simulink model "combined_uc_battery_model"  (R2020a)
settings: Solver=VariableStepAuto  StartTime=0.0  StopTime=3600  RelTol=1e-3
values from neighbouring files (symbols this model uses):
  AH = Q/Vnom    (= 100)    [combined_uc_lion.m]
  Ri = 0.001    [combined_uc_lion.m]
  SOC0 = 0.5    [combined_uc_lion.m]
undefined symbols (not defined in the file or in its folder): DiscIntNeverNeededParam
libraries: fl_lib x5, nesl_utility x4, ee_lib x3
settings Model: Creator=sateeshk  LastModifiedBy=sateeshk

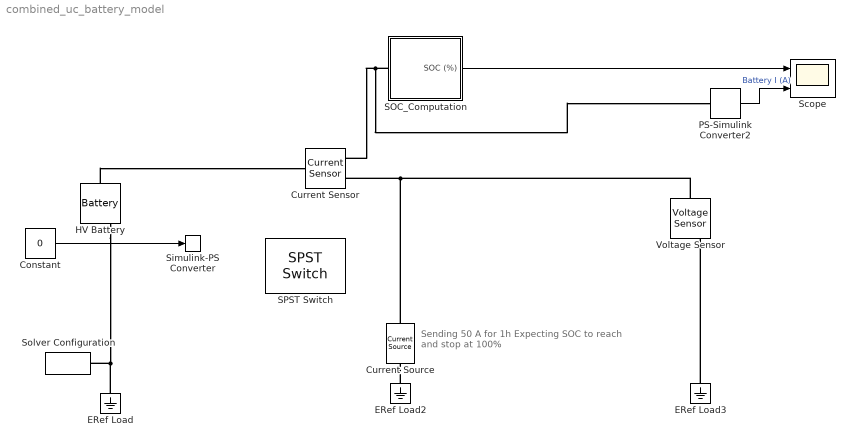
== system combined_uc_battery_model ==
  note: Sending 50 A for 1h
      | Expecting SOC to reach and stop at 100%
  Constant : Constant  Value=0
  Current Sensor : fl_lib/Electrical/Electrical Sensors/Current Sensor
  Current Source : ee_lib/Sources/Current Source  dc_current=50 A  ac_current=0 A  ac_shift=0 rad  ac_frequency=0 Hz  noise_mode=0  PSD=0 A^2/Hz  repeatability=1  auto_seed=4251803758  user_seed=0  sample_time=1e-3 s  i_specify=off  i_priority=None  i=0 A  i_nominal_specify=off  i_nominal_unit=A  i_nominal_value=1  v_specify=off  v_priority=None  v=0 V  v_nominal_specify=off  v_nominal_unit=V  v_nominal_value=1
      settings: SourceProductBaseCode=PS
  ERef Load : fl_lib/Electrical/Electrical Elements/Electrical Reference
      settings: SourceProductBaseCode=MT,SS
  ERef Load2 : fl_lib/Electrical/Electrical Elements/Electrical Reference
      settings: SourceProductBaseCode=MT,SS
  ERef Load3 : fl_lib/Electrical/Electrical Elements/Electrical Reference
      settings: SourceProductBaseCode=MT,SS
  HV Battery : ee_lib/Sources/Battery  Vnom=Vnom V  R1=Ri Ohm  prm_AH=2  AH=AH hr*A  V1=V1 V  AH1=AH1 hr*A  prm_R2=1  R2=2000 Ohm  prm_dyn=1  Rp1=0.005 Ohm  tau1=30 s  Rp2=0.005 Ohm  tau2=30 s  Rp3=0.005 Ohm  tau3=30 s  Rp4=0.005 Ohm  tau4=30 s  Rp5=0.005 Ohm  tau5=30 s  prm_fade=1  N_fade=100  AH_fade=45 hr*A  R1_fade=2.02 Ohm  V1_fade=10.35 V  i_specify=off  i_priority=None  i=0 A  i_nominal_specify=off  i_nominal_unit=A  i_nominal_value=1  v_specify=off  v_priority=None  v=0 V  v_nominal_specify=off  v_nominal_unit=V  v_nominal_value=1  charge_specify=off  charge_priority=High  charge=AH0 hr*A  charge_nominal_specify=off  charge_nominal_unit=hr*A  charge_nominal_value=1  num_cycles_specify=off  num_cycles_priority=High  num_cycles=0  num_cycles_nominal_specify=off  num_cycles_nominal_unit=1  num_cycles_nominal_value=1  thermal_mass=89400 J/K  Tmeas=25 degC  Vnom_T2=Vnom V  R1_T2=Ri+0.1*Ri Ohm  V1_T2=V1 V  R2_T2=2200 Ohm  Rp1_T2=0.005 Ohm  tau1_T2=30 s  Rp2_T2=0.005 Ohm  tau2_T2=30 s  Rp3_T2=0.005 Ohm  tau3_T2=30 s  Rp4_T2=0.005 Ohm  tau4_T2=30 s  Rp5_T2=0.005 Ohm  tau5_T2=30 s  Tmeas2=0 degC  temperature_specify=off  temperature_priority=High  temperature=25 degC  temperature_nominal_specify=off  temperature_nominal_unit=K  temperature_nominal_value=1
      settings: AttributesFormatString=100 Ah  InternalSimscapePortConfiguration="{\"Bottom\":[],\"Left\":[{\"id\":\"p\",\"label\":\"+\",\"type\":\"foundation.electrical.electrical\"}],\"Right\":[{\"id\":\"n\",\"label\":\"-\",\"type\":\"foundation.electrical.electrical\"},{\"id\":\"H\",\"label\":\"H\",\"type\":\"foundation.thermal.thermal\"}],\"Top\":[]}"
  PS-Simulink Converter2 : nesl_utility/PS-Simulink Converter  PhysicalDomain=network_engine_domain  SubClassName=ps_output  LeftPortType=input  RightPortType=output  PseudoPeriodic=off  Frequencies=[]  Unit=1  AffineConversion=off
      settings: SourceProductBaseCode=MT,SS
  SOC_Computation : Subsystem
  SPST Switch : ee_lib/Switches & Breakers/SPST Switch  R_closed=0.01 Ohm  G_open=1e-6 S  Threshold=0.5 V  Width=0 V  model_dynamics=0  t_on=1e-3 s  t_off=1e-3 s  initial_vT=0 V
      settings: SourceProductBaseCode=PS  LogSimulationData=on  InternalSimscapePortConfiguration="{\"Bottom\":[],\"Left\":[{\"id\":\"vT\",\"label\":\"vT\",\"type\":\"input\"},{\"id\":\"p\",\"label\":\"\",\"type\":\"foundation.electrical.electrical\"}],\"Right\":[{\"id\":\"n\",\"label\":\"\",\"type\":\"foundation.electrical.electrical\"}],\"Top\":[]}"
  Scope : Scope  NumInputPorts=2
  Simulink-PS Converter : nesl_utility/Simulink-PS Converter  PhysicalDomain=network_engine_domain  SubClassName=ps_input  LeftPortType=input  RightPortType=output  PseudoPeriodic=off  Frequencies=[]  NoiseDistribution=none  NoiseParameters=[]  Unit=1  AffineConversion=off  FilteringAndDerivatives=provide  SimscapeFilterOrder=1  InputFilterTimeConstant=0.001  UdotUserProvided=0
  Solver Configuration : nesl_utility/Solver Configuration  PhysicalDomain=network_engine_domain  SubClassName=solver  LeftPortType=input  RightPortType=generic  Tones=[]  Harmonics=[]  SimulateNoise=off  Profile=off  UseLocalSampling=off  EnableSwitchedLinearOptims=on  FrequencyDomain=off  UseCCode=off  RelTol=0.001  AbsTol=1e-06  MinStep=1e-09  ToWorkspace=off  RevertToSquareIcSolve=off  NumHomotopyIterations=100  PhasorMode=off  PhasorModeNumHarmonics=1  DoDC=off  ResidualTolerance=1e-9  UseLocalSolver=off  LocalSolverChoice=NE_BACKWARD_EULER_ADVANCER  LocalSolverSampleTime=0.01  DoFixedCost=off  MaxNonlinIter=3  MaxModeIter=2  LinearAlgebra=auto  EquationFormulation=NE_TIME_EF  DelaysMemoryBudget=1024  AutomaticFiltering=on  FilteringTimeConstant=0.001  PartitionStorageMethod=AS_NEEDED  PartitionMemoryBudget=1024  PartitionMethod=FAST
      settings: SourceProductBaseCode=MT,SS
  Voltage Sensor : fl_lib/Electrical/Electrical Sensors/Voltage Sensor
  wires:
  SOC_Computation/1(SOC (%)) -> Scope/1
  PS-Simulink Converter2/1 -> Scope/2  "Battery I (A)"
  Constant/1 -> Simulink-PS Converter/1
  connections:
  ERef Load/LConn1 -- HV Battery/RConn1 -- Solver Configuration/RConn1
  HV Battery/LConn1 -- Current Sensor/LConn1
  SOC_Computation/LConn1 -- PS-Simulink Converter2/LConn1 -- Current Sensor/RConn1
  Voltage Sensor/LConn1 -- Current Source/LConn1 -- Current Sensor/RConn2
  ERef Load3/LConn1 -- Voltage Sensor/RConn2
  ERef Load2/LConn1 -- Current Source/RConn1

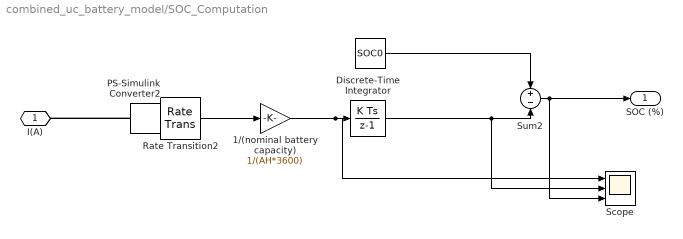
== system combined_uc_battery_model/SOC_Computation ==
  " " : Constant  Value=SOC0
  1/(nominal battery capacity) : Gain  Gain=1/(AH*3600)
  Discrete-Time Integrator : DiscreteIntegrator  SampleTime=-1  ICPrevOutput=DiscIntNeverNeededParam  ICPrevScaledInput=DiscIntNeverNeededParam
  PS-Simulink Converter2 : nesl_utility/PS-Simulink Converter  PhysicalDomain=network_engine_domain  SubClassName=ps_output  LeftPortType=input  RightPortType=output  PseudoPeriodic=off  Frequencies=[]  Unit=A  AffineConversion=off
      settings: SourceProductBaseCode=MT,SS
  Rate Transition2 : RateTransition
  Scope : Scope  NumInputPorts=3
  Sum2 : Sum  Inputs=+-
  I(A) : PMIOPort  Side=Left
  SOC (%) : Outport
  wires:
  Rate Transition2/1 -> 1/(nominal battery capacity)/1
  " "/1 -> Sum2/1
  1/(nominal battery capacity)/1 -> Scope/1, Discrete-Time Integrator/1
  Discrete-Time Integrator/1 -> Scope/2, Sum2/2
  PS-Simulink Converter2/1 -> Rate Transition2/1
  Sum2/1 -> SOC (%)/1, Scope/3
  connections:
  PS-Simulink Converter2/LConn1 -- I(A)/RConn1
